simulink model "HSM_4p6U10_Motion_v01_06022022_NEW_ECC_2019a"  (R2019a)
settings: Solver=ode1  StartTime=0.0  StopTime=Inf  FixedStep=Ts  RelTol=1e-3  EnableMultiTasking=on
PostLoadFcn:
  | , if any(exist('dsrtsu_mdlpostloadfcn', 'file') == [2, 3, 6]), try dsrtsu_mdlpostloadfcn('Execute', bdroot); catch fprintf('Error in PostLoadFcn (dsrtsu_mdlpostloadfcn) for model "%s":\n %s\n', bdroot, lasterr); end, end,
values from neighbouring files (symbols this model uses):
  CDP = -1    [Parameters_4p6U10.m]
  CUP = 1    [Parameters_4p6U10.m]
  HDP = 1    [Parameters_4p6U10.m]
  HUP = -1    [Parameters_4p6U10.m]
  K1m = 1.7E-4    (= 0.00017)    [Parameters_4p6U10.m]
  K2m = 7.0E-4    (= 0.0007)    [Parameters_4p6U10.m]
  Ts = 0.0002    [Parameters_4p6U10.m]
undefined symbols (not defined in the file or in its folder): GPTRIP1SEL, GPTRIP2SEL, TZ1, TZ2
libraries: simulink_extras x25, simulink x17, c2837xDlib x11, c2802xlib x2, idelinklib_common x1
(part 1 of 3)
PreSaveFcn:
  | , if any(exist('dsmpb_private', 'file') == [2, 3, 6]), try, dsmpb_private('dsmpb_mdlclblib', 'PreSave', bdroot); catch, disp(lasterr); end, end,
CloseFcn:
  | , if any(exist('dsmpb_private', 'file') == [2, 3, 6]), try, dsmpb_private('dsmpb_mdlclblib', 'Close', bdroot); catch, disp(lasterr); end, end,
settings Model: DSRTSU_INTERNAL_RTI_VER=500  DSRTSU_INTERNAL_RTI_TYPE=rti1007  DSRTSU_INTERNAL_RTIFPGA=90  DSMPB_DATASERVER_ModelPortLibVersion1=8  DSMPB_DATASERVER_DataServerVersion1=6  DSMPB_DATASERVER_DataServerStreamVersion1=3  SimulationMode=external  ExtModeTrigDuration=8  Creator=Christos  LastModifiedBy=ThermoLift
settings DataIOCC: ReturnWorkspaceOutputs=off
settings OptimizationCC: BlockReduction=off  ConditionallyExecuteInputs=off  DefaultParameterBehavior=Inlined  DefaultUnderspecifiedDataType=single  StrengthReduction=on  PassReuseOutputArgsAs=Individual arguments  MaxStackSize=512  OptimizeBlockOrder=speed
settings DebuggingCC: AlgebraicLoopMsg=none  ArtificialAlgebraicLoopMsg=none  ParameterPrecisionLossMsg=none  ParameterTunabilityLossMsg=error  SFUnexpectedBacktrackingDiag=warning  SFNoUnconditionalDefaultTransitionDiag=warning  SFExecutionAtInitializationDiag=none  ArithmeticOperatorsInVariantConditions=warning
settings HardwareCC: ProdBitPerChar=16  ProdBitPerInt=16  ProdBitPerPointer=32  ProdBitPerSizeT=32  ProdBitPerPtrDiffT=32  ProdLargestAtomicInteger=Integer  ProdLargestAtomicFloat=None  ProdWordSize=16  ProdHWDeviceType=Texas Instruments->C2000  TargetIntDivRoundTo=Zero  TargetEndianess=BigEndian  TargetHWDeviceType=Custom Processor->Custom
settings SFSimCC: SimUseLocalCustomCode=off  MATLABDynamicMemAlloc=off
settings RTWCC: SystemTargetFile=ert.tlc  HardwareBoard=TI Delfino F28379D LaunchPad  TLCOptions=-aInlineSetEventsForThisBaseRateFcn=TLC_FALSE -aSuppressMultiTaskScheduler=TLC_FALSE -aRateBasedStepFcn=1  TemplateMakefile=ert_default_tmf  GenerateReport=on  RTWUseLocalCustomCode=off  Toolchain=Texas Instruments Code Composer Studio (C2000)  IncludeHyperlinkInReport=on  LaunchReport=on  GenerateTraceInfo=on  GenerateTraceReport=on  GenerateTraceReportSl=on  GenerateTraceReportSf=on  GenerateTraceReportEml=on
settings CodeAppCC: ForceParamTrailComments=on  IgnoreCustomStorageClasses=off  OperatorAnnotations=on  SimulinkDataObjDesc=on  SFDataObjDesc=on  InsertBlockDesc=on  StateflowObjectComments=on
settings ERTTargetCC: CodeReplacementLibrary=TI C28x  SupportContinuousTime=on
settings ConfigComp: CovMetricSettings=dw  CovHtmlReporting=on  CovSaveCumulativeToWorkspaceVar=on  CovSaveSingleToWorkspaceVar=on  CovExternalEMLEnable=off
settings SimscapeCC: SimscapeNormalizeSystem=off

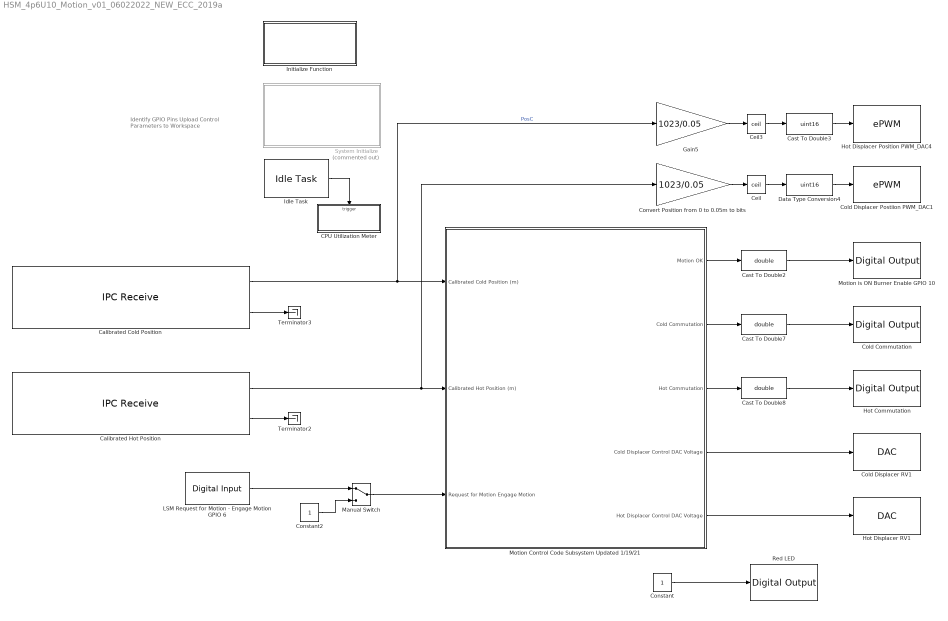
== system HSM_4p6U10_Motion_v01_06022022_NEW_ECC_2019a ==
  note: Identify GPIO Pins
      | Upload Control Parameters to Workspace
  CPU Utilization Meter : Subsystem  TreatAsAtomicUnit=on
  "Calibrated Cold Position " : c2837xDlib/IPC Receive  SelectChannel=0  DataType=single  DataLength=1  EnableBlocking=off  SampleTime=Ts
      settings: SourceProductName=Embedded Coder Support Package for Texas Instruments C2000 Processors  SourceProductBaseCode=TIC2000
  Calibrated Hot Position : c2837xDlib/IPC Receive  SelectChannel=1  DataType=single  DataLength=1  EnableBlocking=off  SampleTime=Ts
      settings: SourceProductName=Embedded Coder Support Package for Texas Instruments C2000 Processors  SourceProductBaseCode=TIC2000
  Cast To Double2 : DataTypeConversion  OutDataTypeStr=double
  Cast To Double3 : DataTypeConversion  OutDataTypeStr=uint16
  Cast To Double7 : DataTypeConversion  OutDataTypeStr=double
  Cast To Double8 : DataTypeConversion  OutDataTypeStr=double
  Ceil : Rounding  Operator=ceil
  Ceil3 : Rounding  Operator=ceil
  Cold Commutation : c2837xDlib/Digital Output  GPIO_Number=GPIO24~GPIO31  GPIO_Bit0=off  GPIO_BIT0_Toggle=off  GPIO_Bit1=off  GPIO_BIT1_Toggle=off  GPIO_Bit2=off  GPIO_BIT2_Toggle=off  GPIO_Bit3=on  GPIO_BIT3_Toggle=off  GPIO_Bit4=off  GPIO_BIT4_Toggle=off  GPIO_Bit5=off  GPIO_BIT5_Toggle=off  GPIO_Bit6=off  GPIO_BIT6_Toggle=off  GPIO_Bit7=off  GPIO_BIT7_Toggle=off
      settings: SourceProductName=Embedded Coder Support Package for Texas Instruments C2000 Processors  SourceProductBaseCode=TIC2000
  Cold Displacer Postiion PWM_DAC1 : c2802xlib/ePWM  useModule=ePWM6  ePWMxLINKTBPRD=Not Linked  periodUnits=Clock cycles  timerSource=Specify via dialog  timerPeriod_clk=1023  timerPeriod_sec=0.0001  tbshadow=Counter equals to zero  countingMode=Up  phaseActiveEnable=Disable  phaseDirection=Count down after sync  phaseActive=0  synchronizationEnable=off  dcaevt1Sync=off  dcbevt1Sync=off  synchronizationOption=Disable  clockPrescale=1  HSclockPrescale=1  enswap=off  ePWMxAStatus=off  ePWMxAactionLogic1=Do nothing  ePWMxAactionLogic2=Set  ePWMxAactionLogic3=Clear  ePWMxAactionLogic4=Set  ePWMxAactionLogic5=Do nothing  ePWMxAactionLogic6=Do nothing  ePWMxALoadMode=Load on counter equals to zero (CTR=Zero)  ePWMxACSFenable=off  ePWMxACSFvalue=Forcing disable  ePWMxASFreload=Zero  ePWMxBStatus=on  ePWMxBactionLogic1=Do nothing  ePWMxBactionLogic2=Set  ePWMxBactionLogic3=Do nothing  ePWMxBactionLogic4=Do nothing  ePWMxBactionLogic5=Clear  ePWMxBactionLogic6=Set  ePWMxBLoadMode=Load on counter equals to zero (CTR=Zero)  ePWMxBCSFenable=off  ePWMxBCSFvalue=Forcing disable  ePWMxBSFreload=Zero  ePWNxBOutWay=off  ePWMxLINKCMPA=Not Linked  CMPAUnits=Clock cycles  CMPASource=Input port  CMPAValue_per=50  CMPAValue_clk=0  enCMPAshadow=Counter equals to zero  ePWMxLINKCMPB=Not Linked  CMPBUnits=Clock cycles  CMPBSource=Specify via dialog  CMPBValue_per=50  CMPBValue_clk=0  enCMPBshadow=Counter equals to zero  ePWMxLINKCMPC=Not Linked  CMPCUnits=Clock cycles  CMPCSource=Specify via dialog  CMPCValue_per=50  CMPCValue_clk=0  enCMPCshadow=Counter equals to zero  ePWMxLINKCMPD=Not Linked  CMPDUnits=Clock cycles  CMPDSource=Specify via dialog  CMPDValue_per=50  CMPDValue_clk=0  enCMPDshadow=Counter equals to zero  enableDBePWMxA=off  enableDBePWMxB=off  enhalfcycle=off  DBpolarity=Active high (AH)  DBedgeDelay=Positive  DBSource_ePWMxA=ePWMxA  DBSource_ePWMxB=ePWMxA  DBperiodSource=Specify via dialog  REDperiod=0  FEDperiod=0  adcstartModuleA=off  adcrequestEventA=First event  adcstartEventA=Digital Compare Module A Event 1 start of conversion (DCAEVT1.soc)  adcstartEventA_type2=Digital Compare Module A Event 1 start of conversion (DCAEVT1.soc)  adcstartModuleB=off  adcrequestEventB=First event  adcstartEventB=Counter equals to zero (CTR=Zero)  adcstartEventB_type2=Counter equals to zero (CTR=Zero)  intEn=off  intPrd=First event  intSel=Counter equals to zero (CTR=Zero)  intSel_type2=Counter equals to zero (CTR=Zero)  hrpe=off  enHRPWM=off  HRPWM_LoadMode=Counter equals to period (CTR=PRD)  HRPWM_CTLMode=Duty or Period control mode  HRPWM_EDGMode=Both edge  hrpeb=off  enHRPWMB=off  HRPWM_LoadModeB=Counter equals to zero (CTR=ZERO)  HRPWM_CTLModeB=Duty or Period control mode  HRPWM_EDGModeB=Both edge  enSFO=on  enautoconv=on  chopperEnable=off  chopperFrequency=1  chopperFirstwidth=1  chopperDuty=12.5%  tripZonesource=Specify via dialog  tzselOSHT1=off  tzselOSHT2=off  tzselOSHT3=off  tzselOSHDCAEV1=off  tzselOSHDCBEV1=off  tzselCBC1=off  tzselCBC2=off  tzselCBC3=off  tzselCBCDCAEV2=off  tzselCBCDCBEV2=off  tzselOSHT4=off  tzselOSHT5=off  tzselOSHT6=off  tzselCBC4=off  tzselCBC5=off  tzselCBC6=off  enTzOstIntr=off  enTzCbcIntr=off  enTzDCAEVT1Intr=off  enTzDCAEVT2Intr=off  enTzDCBEVT1Intr=off  enTzDCBEVT2Intr=off  ePWMxAforced=No action  ePWMxBforced=No action  DCAEVT1forced=No action  DCBEVT1forced=No action  DCAEVT2forced=No action  DCBEVT2forced=No action  dcah=Trip Zone 1 input (TZ1)  dcal=Trip Zone 2 input (TZ2)  dcbh=Trip Zone 1 input (TZ1)  dcbl=Trip Zone 2 input (TZ2)  dcah_type2=GPTRIP1SEL/(TZ1)  dcal_type2=GPTRIP2SEL/(TZ2)  dcbh_type2=GPTRIP1SEL/(TZ1)  dcbl_type2=GPTRIP2SEL/(TZ2)  gendcaevt1=Event disabled  gendcaevt2=Event disabled  gendcbevt1=Event disabled  gendcbevt2=Event disabled  dcaevt1src=DCAEVT1 with sync  dcaevt2src=DCAEVT2 with sync  dcbevt1src=DCBEVT1 with sync  dcbevt2src=DCBEVT2 with sync  pulsesel=Counter equals to zero (CTR=Zero)  blankinv=off  blankoffset=0  blankwidth=0  evsrcsel=Filtered version of DCAEVT1 (DCAEVT1FILT)  encape=off  PwmType=C2000_Type4
      settings: SourceProductName=Embedded Coder Support Package for Texas Instruments C2000 Processors
  Cold Displacer RV1 : c2837xDlib/DAC  channel=B  saturate=on
      settings: SourceProductName=Embedded Coder Support Package for Texas Instruments C2000 Processors  SourceProductBaseCode=TIC2000
  Constant : Constant  OutDataTypeStr=boolean
  Constant2 : Constant  OutDataTypeStr=boolean
  Convert Position from 0 to 0.05m to bits : Gain  Gain=1023/0.05
  Data Type Conversion4 : DataTypeConversion  OutDataTypeStr=uint16
  Gain5 : Gain  Gain=1023/0.05
  Hot Commutation : c2837xDlib/Digital Output  GPIO_Number=GPIO24~GPIO31  GPIO_Bit0=off  GPIO_BIT0_Toggle=off  GPIO_Bit1=on  GPIO_BIT1_Toggle=off  GPIO_Bit2=off  GPIO_BIT2_Toggle=off  GPIO_Bit3=off  GPIO_BIT3_Toggle=off  GPIO_Bit4=off  GPIO_BIT4_Toggle=off  GPIO_Bit5=off  GPIO_BIT5_Toggle=off  GPIO_Bit6=off  GPIO_BIT6_Toggle=off  GPIO_Bit7=off  GPIO_BIT7_Toggle=off
      settings: SourceProductName=Embedded Coder Support Package for Texas Instruments C2000 Processors  SourceProductBaseCode=TIC2000
  Hot Displacer Position PWM_DAC4 : c2802xlib/ePWM  useModule=ePWM5  ePWMxLINKTBPRD=Not Linked  periodUnits=Clock cycles  timerSource=Specify via dialog  timerPeriod_clk=1023  timerPeriod_sec=0.0001  tbshadow=Counter equals to zero  countingMode=Up  phaseActiveEnable=Disable  phaseDirection=Count down after sync  phaseActive=0  synchronizationEnable=off  dcaevt1Sync=off  dcbevt1Sync=off  synchronizationOption=Disable  clockPrescale=1  HSclockPrescale=1  enswap=off  ePWMxAStatus=on  ePWMxAactionLogic1=Do nothing  ePWMxAactionLogic2=Set  ePWMxAactionLogic3=Clear  ePWMxAactionLogic4=Set  ePWMxAactionLogic5=Do nothing  ePWMxAactionLogic6=Do nothing  ePWMxALoadMode=Load on counter equals to zero (CTR=Zero)  ePWMxACSFenable=off  ePWMxACSFvalue=Forcing disable  ePWMxASFreload=Zero  ePWMxBStatus=off  ePWMxBactionLogic1=Do nothing  ePWMxBactionLogic2=Set  ePWMxBactionLogic3=Do nothing  ePWMxBactionLogic4=Do nothing  ePWMxBactionLogic5=Clear  ePWMxBactionLogic6=Set  ePWMxBLoadMode=Load on counter equals to zero (CTR=Zero)  ePWMxBCSFenable=off  ePWMxBCSFvalue=Forcing disable  ePWMxBSFreload=Zero  ePWNxBOutWay=off  ePWMxLINKCMPA=Not Linked  CMPAUnits=Clock cycles  CMPASource=Specify via dialog  CMPAValue_per=50  CMPAValue_clk=0  enCMPAshadow=Counter equals to zero  ePWMxLINKCMPB=Not Linked  CMPBUnits=Clock cycles  CMPBSource=Input port  CMPBValue_per=50  CMPBValue_clk=0  enCMPBshadow=Counter equals to zero  ePWMxLINKCMPC=Not Linked  CMPCUnits=Clock cycles  CMPCSource=Specify via dialog  CMPCValue_per=50  CMPCValue_clk=0  enCMPCshadow=Counter equals to zero  ePWMxLINKCMPD=Not Linked  CMPDUnits=Clock cycles  CMPDSource=Specify via dialog  CMPDValue_per=50  CMPDValue_clk=0  enCMPDshadow=Counter equals to zero  enableDBePWMxA=off  enableDBePWMxB=off  enhalfcycle=off  DBpolarity=Active high (AH)  DBedgeDelay=Positive  DBSource_ePWMxA=ePWMxA  DBSource_ePWMxB=ePWMxA  DBperiodSource=Specify via dialog  REDperiod=0  FEDperiod=0  adcstartModuleA=off  adcrequestEventA=First event  adcstartEventA=Digital Compare Module A Event 1 start of conversion (DCAEVT1.soc)  adcstartEventA_type2=Digital Compare Module A Event 1 start of conversion (DCAEVT1.soc)  adcstartModuleB=off  adcrequestEventB=First event  adcstartEventB=Counter equals to zero (CTR=Zero)  adcstartEventB_type2=Counter equals to zero (CTR=Zero)  intEn=off  intPrd=First event  intSel=Counter equals to zero (CTR=Zero)  intSel_type2=Counter equals to zero (CTR=Zero)  hrpe=off  enHRPWM=off  HRPWM_LoadMode=Counter equals to period (CTR=PRD)  HRPWM_CTLMode=Duty or Period control mode  HRPWM_EDGMode=Both edge  hrpeb=off  enHRPWMB=off  HRPWM_LoadModeB=Counter equals to zero (CTR=ZERO)  HRPWM_CTLModeB=Duty or Period control mode  HRPWM_EDGModeB=Both edge  enSFO=on  enautoconv=on  chopperEnable=off  chopperFrequency=1  chopperFirstwidth=1  chopperDuty=12.5%  tripZonesource=Specify via dialog  tzselOSHT1=off  tzselOSHT2=off  tzselOSHT3=off  tzselOSHDCAEV1=off  tzselOSHDCBEV1=off  tzselCBC1=off  tzselCBC2=off  tzselCBC3=off  tzselCBCDCAEV2=off  tzselCBCDCBEV2=off  tzselOSHT4=off  tzselOSHT5=off  tzselOSHT6=off  tzselCBC4=off  tzselCBC5=off  tzselCBC6=off  enTzOstIntr=off  enTzCbcIntr=off  enTzDCAEVT1Intr=off  enTzDCAEVT2Intr=off  enTzDCBEVT1Intr=off  enTzDCBEVT2Intr=off  ePWMxAforced=No action  ePWMxBforced=No action  DCAEVT1forced=No action  DCBEVT1forced=No action  DCAEVT2forced=No action  DCBEVT2forced=No action  dcah=Trip Zone 1 input (TZ1)  dcal=Trip Zone 2 input (TZ2)  dcbh=Trip Zone 1 input (TZ1)  dcbl=Trip Zone 2 input (TZ2)  dcah_type2=GPTRIP1SEL/(TZ1)  dcal_type2=GPTRIP2SEL/(TZ2)  dcbh_type2=GPTRIP1SEL/(TZ1)  dcbl_type2=GPTRIP2SEL/(TZ2)  gendcaevt1=Event disabled  gendcaevt2=Event disabled  gendcbevt1=Event disabled  gendcbevt2=Event disabled  dcaevt1src=DCAEVT1 with sync  dcaevt2src=DCAEVT2 with sync  dcbevt1src=DCBEVT1 with sync  dcbevt2src=DCBEVT2 with sync  pulsesel=Counter equals to zero (CTR=Zero)  blankinv=off  blankoffset=0  blankwidth=0  evsrcsel=Filtered version of DCAEVT1 (DCAEVT1FILT)  encape=off  PwmType=C2000_Type4
      settings: SourceProductName=Embedded Coder Support Package for Texas Instruments C2000 Processors
  Hot Displacer RV1 : c2837xDlib/DAC  channel=A  saturate=on
      settings: SourceProductName=Embedded Coder Support Package for Texas Instruments C2000 Processors  SourceProductBaseCode=TIC2000
  Idle Task : idelinklib_common/Idle Task  tasknumbers=[1]  taskpriorities=100017  taskpreempts=[1]  showinput=off  simPriority=0
      settings: SourceProductName=MATLAB Coder  SourceProductBaseCode=ME
  Initialize Function : Subsystem  TreatAsAtomicUnit=on
  LSM Request for Motion - Engage Motion GPIO 6 : c2837xDlib/Digital Input  GPIO_Number=GPIO0~GPIO7  GPIO_Bit0=off  GPIO_Bit1=off  GPIO_Bit2=off  GPIO_Bit3=off  GPIO_Bit4=off  GPIO_Bit5=off  GPIO_Bit6=on  GPIO_Bit7=off  sampleTime=Ts  dataType=boolean  GPIO_Bit0_Qualification=Sync to SYSCLKOUT  GPIO_Bit1_Qualification=Sync to SYSCLKOUT  GPIO_Bit2_Qualification=Sync to SYSCLKOUT  GPIO_Bit3_Qualification=Sync to SYSCLKOUT  GPIO_Bit4_Qualification=Sync to SYSCLKOUT  GPIO_Bit5_Qualification=Sync to SYSCLKOUT  GPIO_Bit6_Qualification=Sync to SYSCLKOUT  GPIO_Bit7_Qualification=Sync to SYSCLKOUT  Qualification_Period=-1
      settings: SourceProductName=Embedded Coder Support Package for Texas Instruments C2000 Processors  SourceProductBaseCode=TIC2000
  Manual Switch : ManualSwitch
  Motion Control Code Subsystem Updated 1/19/21 : Subsystem
  Motion is ON Burner Enable GPIO 10 : c2837xDlib/Digital Output  GPIO_Number=GPIO8~GPIO15  GPIO_Bit0=off  GPIO_BIT0_Toggle=off  GPIO_Bit1=off  GPIO_BIT1_Toggle=off  GPIO_Bit2=on  GPIO_BIT2_Toggle=off  GPIO_Bit3=off  GPIO_BIT3_Toggle=off  GPIO_Bit4=off  GPIO_BIT4_Toggle=off  GPIO_Bit5=off  GPIO_BIT5_Toggle=off  GPIO_Bit6=off  GPIO_BIT6_Toggle=off  GPIO_Bit7=off  GPIO_BIT7_Toggle=off
      settings: SourceProductName=Embedded Coder Support Package for Texas Instruments C2000 Processors  SourceProductBaseCode=TIC2000
  Red LED : c2837xDlib/Digital Output  GPIO_Number=GPIO120~GPIO127  GPIO_Bit0=off  GPIO_BIT0_Toggle=off  GPIO_Bit1=off  GPIO_BIT1_Toggle=off  GPIO_Bit2=on  GPIO_BIT2_Toggle=off  GPIO_Bit3=off  GPIO_BIT3_Toggle=off  GPIO_Bit4=off  GPIO_BIT4_Toggle=off  GPIO_Bit5=off  GPIO_BIT5_Toggle=off  GPIO_Bit6=off  GPIO_BIT6_Toggle=off  GPIO_Bit7=off  GPIO_BIT7_Toggle=off
      settings: SourceProductName=Embedded Coder Support Package for Texas Instruments C2000 Processors  SourceProductBaseCode=TIC2000
  System Initialize : Subsystem  Commented=on  mask(System Initialize){ShowInLibBrowser=0}
      mask prompts: ShowInLibBrowser "Simulink:masks:CustCodeMaskParam1_MP"
      settings: CopyFcn=cccopyfcn(gcb)  OpenFcn=ccopenfcn('System Initialize Function')
      mask Help: eval('feval(''rtwprivate'',''rtwhelpview'',''rtw_sys_initialize_block'')');
      mask Display: disp('System\nInitialize');
  Terminator2 : Terminator
  Terminator3 : Terminator
  wires:
  Idle Task/1 -> CPU Utilization Meter/Trigger
  "Calibrated Cold Position "/2 -> Terminator3/1
  Calibrated Hot Position/2 -> Terminator2/1
  "Calibrated Cold Position "/1 -> Gain5/1, Motion Control Code Subsystem Updated 1/19/21/1(Calibrated Cold Position (m))  "PosC"
  Motion Control Code Subsystem Updated 1/19/21/2(Cold Commutation) -> Cast To Double7/1
  Cast To Double3/1 -> Hot Displacer Position PWM_DAC4/1
  Convert Position from 0 to 0.05m to bits/1 -> Ceil/1
  Ceil3/1 -> Cast To Double3/1
  Ceil/1 -> Data Type Conversion4/1
  Data Type Conversion4/1 -> Cold Displacer Postiion PWM_DAC1/1
  Cast To Double7/1 -> Cold Commutation/1
  Motion Control Code Subsystem Updated 1/19/21/4(Cold Displacer Control DAC Voltage) -> Cold Displacer RV1/1
  Gain5/1 -> Ceil3/1
  Motion Control Code Subsystem Updated 1/19/21/1(Motion OK) -> Cast To Double2/1
  Cast To Double2/1 -> Motion is ON Burner Enable GPIO 10/1
  Motion Control Code Subsystem Updated 1/19/21/3(Hot Commutation) -> Cast To Double8/1
  Motion Control Code Subsystem Updated 1/19/21/5(Hot Displacer Control DAC Voltage) -> Hot Displacer RV1/1
  Cast To Double8/1 -> Hot Commutation/1
  Constant/1 -> Red LED/1
  Calibrated Hot Position/1 -> Convert Position from 0 to 0.05m to bits/1, Motion Control Code Subsystem Updated 1/19/21/2(Calibrated Hot Position (m))
  LSM Request for Motion - Engage Motion GPIO 6/1 -> Manual Switch/1
  Constant2/1 -> Manual Switch/2
  Manual Switch/1 -> Motion Control Code Subsystem Updated 1/19/21/3(Request for Motion Engage Motion)

== system HSM_4p6U10_Motion_v01_06022022_NEW_ECC_2019a/CPU Utilization Meter ==
  function : TriggerPort  TriggerType=function-call  VariantControl=Variant
  Avg. voltage toggle : c2837xDlib/Digital Output  GPIO_Number=GPIO16~GPIO23  GPIO_Bit0=off  GPIO_BIT0_Toggle=off  GPIO_Bit1=off  GPIO_BIT1_Toggle=on  GPIO_Bit2=off  GPIO_BIT2_Toggle=off  GPIO_Bit3=off  GPIO_BIT3_Toggle=off  GPIO_Bit4=off  GPIO_BIT4_Toggle=off  GPIO_Bit5=off  GPIO_BIT5_Toggle=off  GPIO_Bit6=on  GPIO_BIT6_Toggle=on  GPIO_Bit7=off  GPIO_BIT7_Toggle=off
      settings: SourceProductName=Embedded Coder Support Package for Texas Instruments C2000 Processors  SourceProductBaseCode=TIC2000
  toggle enable : Constant
  wires:
  toggle enable/1 -> Avg. voltage toggle/1

== system HSM_4p6U10_Motion_v01_06022022_NEW_ECC_2019a/Initialize Function ==
  Constant : Constant  OutDataTypeStr=boolean
  Enable Position Sensor Power : c2837xDlib/Digital Output  GPIO_Number=GPIO120~GPIO127  GPIO_Bit0=off  GPIO_BIT0_Toggle=off  GPIO_Bit1=off  GPIO_BIT1_Toggle=off  GPIO_Bit2=on  GPIO_BIT2_Toggle=off  GPIO_Bit3=off  GPIO_BIT3_Toggle=off  GPIO_Bit4=off  GPIO_BIT4_Toggle=off  GPIO_Bit5=off  GPIO_BIT5_Toggle=off  GPIO_Bit6=off  GPIO_BIT6_Toggle=off  GPIO_Bit7=off  GPIO_BIT7_Toggle=off
      settings: SourceProductName=Embedded Coder Support Package for Texas Instruments C2000 Processors  SourceProductBaseCode=TIC2000
  Event Listener : EventListener  DisableCoverage=on  EventName=reset
  wires:
  Constant/1 -> Enable Position Sensor Power/1

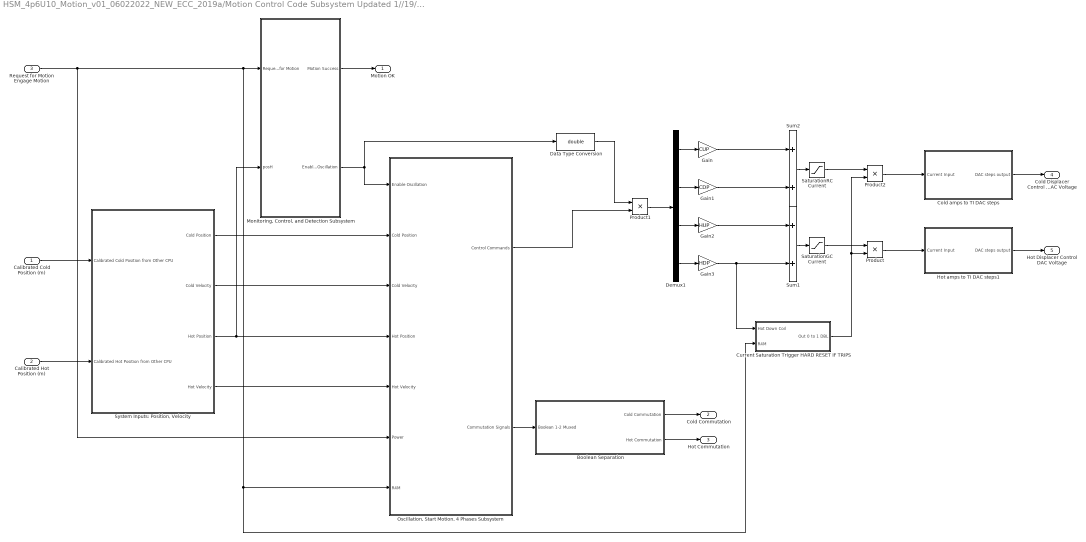
== system HSM_4p6U10_Motion_v01_06022022_NEW_ECC_2019a/Motion Control Code Subsystem Updated 1//19//21 ==
  Calibrated Cold Position (m) : Inport
  Calibrated Hot Position (m) : Inport  Port=2
  Request for Motion Engage Motion : Inport  Port=3
  Boolean Separation : Subsystem
  Cold amps to TI DAC steps : Subsystem
  Current Saturation Trigger HARD RESET IF TRIPS : Subsystem
  Data Type Conversion : DataTypeConversion  OutDataTypeStr=double
  Demux1 : Demux
  Gain : Gain  Gain=CUP
  Gain1 : Gain  Gain=CDP
  Gain2 : Gain  Gain=HUP
  Gain3 : Gain  Gain=HDP
  Hot amps to TI DAC steps1 : Subsystem
  "Monitoring, Control, and Detection Subsystem" : Subsystem
  "Oscillation, Start Motion, 4 Phases Subsystem" : Subsystem
  Product : Product
  Product1 : Product
  Product2 : Product
  SaturationGC Current : Saturate  UpperLimit=40  LowerLimit=-40
  SaturationRC Current : Saturate  UpperLimit=40  LowerLimit=-40
  Sum1 : Sum
  Sum2 : Sum
  "System Inputs: Position, Velocity" : Subsystem
  Motion OK : Outport
  Cold Commutation : Outport  Port=2
  Hot Commutation : Outport  Port=3
  Cold Displacer Control DAC Voltage : Outport  Port=4
  Hot Displacer Control DAC Voltage : Outport  Port=5
  wires:
  "Oscillation, Start Motion, 4 Phases Subsystem"/2(Commutation Signals) -> Boolean Separation/1(Boolean 1-2 Muxed)
  Calibrated Cold Position (m)/1 -> "System Inputs: Position, Velocity"/1(Calibrated Cold Position from Other CPU)
  Calibrated Hot Position (m)/1 -> "System Inputs: Position, Velocity"/2(Calibrated Hot Position from Other CPU)
  "Monitoring, Control, and Detection Subsystem"/2(Enable Oscillation) -> "Oscillation, Start Motion, 4 Phases Subsystem"/1("Enable Oscillation "), Data Type Conversion/1
  Boolean Separation/1(Cold Commutation) -> Cold Commutation/1
  Boolean Separation/2(Hot Commutation) -> Hot Commutation/1
  Hot amps to TI DAC steps1/1(DAC steps output) -> Hot Displacer Control DAC Voltage/1
  Cold amps to TI DAC steps/1("DAC steps output    ") -> Cold Displacer Control DAC Voltage/1
  "System Inputs: Position, Velocity"/1(Cold Position) -> "Oscillation, Start Motion, 4 Phases Subsystem"/2(Cold Position)
  "System Inputs: Position, Velocity"/2(Cold Velocity) -> "Oscillation, Start Motion, 4 Phases Subsystem"/3(Cold Velocity)
  "System Inputs: Position, Velocity"/3(Hot Position) -> "Oscillation, Start Motion, 4 Phases Subsystem"/4(Hot Position), "Monitoring, Control, and Detection Subsystem"/2(posH)
  "System Inputs: Position, Velocity"/4(Hot Velocity) -> "Oscillation, Start Motion, 4 Phases Subsystem"/5(Hot Velocity)
  Request for Motion Engage Motion/1 -> "Oscillation, Start Motion, 4 Phases Subsystem"/6(Power), "Oscillation, Start Motion, 4 Phases Subsystem"/7(R4M), Current Saturation Trigger HARD RESET IF TRIPS/2(R4M), "Monitoring, Control, and Detection Subsystem"/1(Request for Motion)
  "Oscillation, Start Motion, 4 Phases Subsystem"/1("Control Commands ") -> Product1/2
  Data Type Conversion/1 -> Product1/1
  "Monitoring, Control, and Detection Subsystem"/1(Motion Success) -> Motion OK/1
  Current Saturation Trigger HARD RESET IF TRIPS/1(Out 0 to 1 DBL) -> Product2/2, Product/2
  Demux1/2 -> Gain1/1
  Product1/1 -> Demux1/1
  Product/1 -> Hot amps to TI DAC steps1/1(Current Input)
  Gain/1 -> Sum2/1
  SaturationRC Current/1 -> Product2/1
  Product2/1 -> Cold amps to TI DAC steps/1(Current Input)
  Gain2/1 -> Sum1/1
  Sum1/1 -> SaturationGC Current/1
  Demux1/1 -> Gain/1
  Gain3/1 -> Sum1/2, Current Saturation Trigger HARD RESET IF TRIPS/1(Hot Down Coil)
  SaturationGC Current/1 -> Product/1
  Sum2/1 -> SaturationRC Current/1
  Gain1/1 -> Sum2/2
  Demux1/3 -> Gain2/1
  Demux1/4 -> Gain3/1

== system HSM_4p6U10_Motion_v01_06022022_NEW_ECC_2019a/System Initialize ==

== system HSM_4p6U10_Motion_v01_06022022_NEW_ECC_2019a/Motion Control Code Subsystem Updated 1//19//21/Boolean Separation ==
  Boolean 1-2 Muxed : Inport
  Data Type Conversion : DataTypeConversion  OutDataTypeStr=double
  Data Type Conversion1 : DataTypeConversion  OutDataTypeStr=double
  Demux : Demux  Outputs=2
  Gain : Gain  Gain=5
  Gain1 : Gain  Gain=5
  Cold Commutation : Outport
  Hot Commutation : Outport  Port=2
  wires:
  Demux/1 -> Data Type Conversion/1  "Q1Sep"
  Demux/2 -> Data Type Conversion1/1  "Q2Sep"
  Boolean 1-2 Muxed/1 -> Demux/1
  Data Type Conversion/1 -> Gain/1
  Data Type Conversion1/1 -> Gain1/1
  Gain/1 -> Cold Commutation/1
  Gain1/1 -> Hot Commutation/1

== system HSM_4p6U10_Motion_v01_06022022_NEW_ECC_2019a/Motion Control Code Subsystem Updated 1//19//21/Cold amps to TI DAC steps ==
  Current Input : Inport
  Add : Sum
  Amps to Voltage Servo Conversion Gain : Gain  Gain=1/6
  Shift 0 A to DAC midrange : Constant  Value=2098
  Volts to DAC steps : Gain  Gain=208.7
  "DAC steps output    " : Outport
  wires:
  Shift 0 A to DAC midrange/1 -> Add/1
  Volts to DAC steps/1 -> Add/2
  Current Input/1 -> Amps to Voltage Servo Conversion Gain/1
  Add/1 -> "DAC steps output    "/1
  Amps to Voltage Servo Conversion Gain/1 -> Volts to DAC steps/1

== system HSM_4p6U10_Motion_v01_06022022_NEW_ECC_2019a/Motion Control Code Subsystem Updated 1//19//21/Current Saturation Trigger HARD RESET IF TRIPS ==
  Hot Down Coil : Inport
  R4M : Inport  Port=2
  39p5Amps : HitCross  HitCrossingOffset=39.5  HitCrossingDirection=falling
  39p99Amps : HitCross  HitCrossingOffset=39.99  HitCrossingDirection=rising
  Abs : Abs
  Constant : Constant  OutDataTypeStr=double
  Data Type Conversion1 : DataTypeConversion  OutDataTypeStr=double
  Detect Decrease : simulink/Logic and Bit Operations/Detect Decrease  vinit=0.0  OutDataTypeStr=boolean
  Detect Increase : simulink/Logic and Bit Operations/Detect Increase  vinit=0.0  OutDataTypeStr=boolean
  Logical Operator8 : Logic  Operator=NOT  AllPortsSameDT=off  OutDataTypeStr=boolean
  Manual Switch : ManualSwitch  CurrentSetting=0
  Reset : Subsystem
  S-R Flip-Flop : simulink_extras/Flip Flops/S-R Flip-Flop  initial_condition=0
  S-R Flip-Flop1 : simulink_extras/Flip Flops/S-R Flip-Flop  initial_condition=0
  S-R Flip-Flop2 : simulink_extras/Flip Flops/S-R Flip-Flop  initial_condition=0
  Sat Limit : simulink/Logic and Bit Operations/Compare To Constant  relop=>  const=2  OutDataTypeStr=boolean
  Terminator : Terminator
  Terminator1 : Terminator
  Terminator2 : Terminator
  Timer : Subsystem
  Out 0 to 1 DBL : Outport
  wires:
  S-R Flip-Flop1/1 -> Logical Operator8/1
  S-R Flip-Flop/2 -> Terminator1/1
  Logical Operator8/1 -> Data Type Conversion1/1
  Sat Limit/1 -> S-R Flip-Flop1/1  "Coil Timing Trigger"
  39p5Amps/1 -> S-R Flip-Flop/2
  S-R Flip-Flop/1 -> Timer/Enable
  Hot Down Coil/1 -> Abs/1
  39p99Amps/1 -> S-R Flip-Flop/1
  Timer/1(CST) -> Sat Limit/1
  S-R Flip-Flop1/2 -> Terminator2/1
  Data Type Conversion1/1 -> Manual Switch/2
  Abs/1 -> 39p99Amps/1, 39p5Amps/1
  Manual Switch/1 -> Out 0 to 1 DBL/1
  Constant/1 -> Manual Switch/1
  R4M/1 -> Detect Decrease/1, Detect Increase/1
  Detect Increase/1 -> S-R Flip-Flop2/1
  Detect Decrease/1 -> S-R Flip-Flop2/2
  S-R Flip-Flop2/1 -> Reset/Enable
  S-R Flip-Flop2/2 -> Terminator/1
  Reset/1(Reset 2s) -> S-R Flip-Flop1/2

== system HSM_4p6U10_Motion_v01_06022022_NEW_ECC_2019a/Motion Control Code Subsystem Updated 1//19//21/Hot amps to TI DAC steps1 ==
  Current Input : Inport
  Add : Sum
  Amps to Volts Servo Conversion Gain : Gain  Gain=1/6
  Shift 0 A to DAC midrange : Constant  Value=2099
  Volts to DAC steps : Gain  Gain=210
  DAC steps output : Outport
  wires:
  Volts to DAC steps/1 -> Add/2
  Current Input/1 -> Amps to Volts Servo Conversion Gain/1
  Shift 0 A to DAC midrange/1 -> Add/1
  Add/1 -> DAC steps output/1
  Amps to Volts Servo Conversion Gain/1 -> Volts to DAC steps/1

== system HSM_4p6U10_Motion_v01_06022022_NEW_ECC_2019a/Motion Control Code Subsystem Updated 1//19//21/Monitoring, Control, and Detection Subsystem ==
  Request for Motion : Inport
  posH : Inport  Port=2
  Logical Operator2 : Logic  Operator=NOT  AllPortsSameDT=off  OutDataTypeStr=boolean
  Logical Operator5 : Logic  Operator=OR  AllPortsSameDT=off  OutDataTypeStr=boolean
  S-R Flip-Flop : simulink_extras/Flip Flops/S-R Flip-Flop  initial_condition=0
  S-R Flip-Flop1 : simulink_extras/Flip Flops/S-R Flip-Flop  initial_condition=0
  S-R Flip-Flop2 : simulink_extras/Flip Flops/S-R Flip-Flop  initial_condition=0
  Subsystem : Subsystem
  Terminator1 : Terminator
  Terminator3 : Terminator
  Terminator5 : Terminator
  Unit Delay : UnitDelay  SampleTime=-1  HasFrameUpgradeWarning=on
  Unit Delay1 : UnitDelay  SampleTime=-1  HasFrameUpgradeWarning=on
  Motion Success : Outport
  Enable Oscillation : Outport  Port=2
  wires:
  Unit Delay1/1 -> S-R Flip-Flop1/2
  S-R Flip-Flop2/2 -> Terminator1/1
  S-R Flip-Flop2/1 -> Logical Operator5/2
  Logical Operator2/1 -> Logical Operator5/1, S-R Flip-Flop2/2, Unit Delay/1
  Subsystem/1(Motion Failure) -> S-R Flip-Flop2/1
  posH/1 -> Subsystem/2(posH)
  S-R Flip-Flop1/1 -> Motion Success/1  "Enable Start Up Part 1"
  S-R Flip-Flop/1 -> Enable Oscillation/1  "Activate Hot Oscillation,  Attempt to move  Cold Displacer toward BDC"
  Subsystem/2(Motion Success) -> S-R Flip-Flop1/1
  Request for Motion/1 -> S-R Flip-Flop/1, Subsystem/1(Power), Subsystem/3(En Osc), Logical Operator2/1
  Logical Operator5/1 -> Unit Delay1/1
  Unit Delay/1 -> S-R Flip-Flop/2
  S-R Flip-Flop/2 -> Terminator5/1
  S-R Flip-Flop1/2 -> Terminator3/1

== system HSM_4p6U10_Motion_v01_06022022_NEW_ECC_2019a/Motion Control Code Subsystem Updated 1//19//21/Oscillation, Start Motion, 4 Phases Subsystem ==
  "Enable Oscillation " : Inport
  Cold Position : Inport  Port=2
  Cold Velocity : Inport  Port=3
  Hot Position : Inport  Port=4
  Hot Velocity : Inport  Port=5
  Power : Inport  Port=6
  R4M : Inport  Port=7
  Constant : Constant  Value=0  OutDataTypeStr=boolean
  Oscillations Subsystem Time pc No Cold Damping : Subsystem
  Unit Delay : UnitDelay  SampleTime=-1  HasFrameUpgradeWarning=on
  "Control Commands " : Outport
  Commutation Signals : Outport  Port=2
  wires:
  Cold Velocity/1 -> Oscillations Subsystem Time pc No Cold Damping/5(VelC)
  Hot Velocity/1 -> Oscillations Subsystem Time pc No Cold Damping/2(VelH)
  Power/1 -> Oscillations Subsystem Time pc No Cold Damping/3(On/Off)
  Cold Position/1 -> Oscillations Subsystem Time pc No Cold Damping/4(Posc)
  Hot Position/1 -> Oscillations Subsystem Time pc No Cold Damping/1(Hot Position)
  Constant/1 -> Unit Delay/1
  R4M/1 -> Oscillations Subsystem Time pc No Cold Damping/7(R4M)
  "Enable Oscillation "/1 -> Oscillations Subsystem Time pc No Cold Damping/Enable
  Unit Delay/1 -> Oscillations Subsystem Time pc No Cold Damping/6(Enable 4 Phases)
  Oscillations Subsystem Time pc No Cold Damping/2(Commutation Signals) -> Commutation Signals/1
  Oscillations Subsystem Time pc No Cold Damping/1(Control Commands) -> "Control Commands "/1

== system HSM_4p6U10_Motion_v01_06022022_NEW_ECC_2019a/Motion Control Code Subsystem Updated 1//19//21/System Inputs: Position, Velocity ==
  Calibrated Cold Position from Other CPU : Inport
  Calibrated Hot Position from Other CPU : Inport  Port=2
  Cast To Double3 : DataTypeConversion  OutDataTypeStr=double
  Cast To Double4 : DataTypeConversion  OutDataTypeStr=double
  Divide by Ts : Gain  Gain=1/Ts
  Divide by Ts1 : Gain  Gain=1/Ts
  Saturation Cold Velocity : Saturate  UpperLimit=2.2  LowerLimit=-2.2
  Saturation Hot Velocity : Saturate  UpperLimit=2.2  LowerLimit=-2.2
  Second Order Cold Velocity Filter : TransferFcn  Denominator=[9e-8 6e-4 1 ]
  Second Order Hot Velocity Filter : TransferFcn  Denominator=[9e-8 6e-4 1 ]
  Sum2 : Sum  Inputs=+-
  Sum3 : Sum  Inputs=+-
  Unit Delay : UnitDelay  SampleTime=-1  HasFrameUpgradeWarning=on
  Unit Delay1 : UnitDelay  SampleTime=-1  HasFrameUpgradeWarning=on
  Cold Position : Outport
  Cold Velocity : Outport  Port=2
  Hot Position : Outport  Port=3
  Hot Velocity : Outport  Port=4
  wires:
  Calibrated Cold Position from Other CPU/1 -> Cast To Double3/1  "Cold_Position"
  Calibrated Hot Position from Other CPU/1 -> Cast To Double4/1  "Hot_Position"
  Unit Delay/1 -> Sum2/2
  Sum2/1 -> Divide by Ts/1
  Sum3/1 -> Divide by Ts1/1
  Divide by Ts/1 -> Second Order Cold Velocity Filter/1  "Discrete Derivative (Xt+1-Xt)/Ts"
  Saturation Cold Velocity/1 -> Cold Velocity/1  "Cold_Vel"
  Saturation Hot Velocity/1 -> Hot Velocity/1  "Hot_Vel"
  Second Order Cold Velocity Filter/1 -> Saturation Cold Velocity/1
  Second Order Hot Velocity Filter/1 -> Saturation Hot Velocity/1
  Unit Delay1/1 -> Sum3/2
  Divide by Ts1/1 -> Second Order Hot Velocity Filter/1
  Cast To Double3/1 -> Cold Position/1, Unit Delay/1, Sum2/1
  Cast To Double4/1 -> Unit Delay1/1, Hot Position/1, Sum3/1

== system HSM_4p6U10_Motion_v01_06022022_NEW_ECC_2019a/Motion Control Code Subsystem Updated 1//19//21/Current Saturation Trigger HARD RESET IF TRIPS/Reset ==
  Enable : EnablePort  StatesWhenEnabling=reset  ShowOutputPort=on
  Compare To Constant : simulink/Logic and Bit Operations/Compare To Constant  relop=<  const=2  OutDataTypeStr=boolean
  Constant : Constant
  Integrator : Integrator  ExternalReset=rising  LimitOutput=on  UpperSaturationLimit=5
  Reset 2s : Outport
  wires:
  Enable/1 -> Integrator/2
  Integrator/1 -> Compare To Constant/1
  Constant/1 -> Integrator/1
  Compare To Constant/1 -> Reset 2s/1

== system HSM_4p6U10_Motion_v01_06022022_NEW_ECC_2019a/Motion Control Code Subsystem Updated 1//19//21/Current Saturation Trigger HARD RESET IF TRIPS/Timer ==
  Enable : EnablePort  StatesWhenEnabling=reset  ShowOutputPort=on
  Constant : Constant
  Integrator : Integrator  ExternalReset=rising  LimitOutput=on  UpperSaturationLimit=2
  CST : Outport
  wires:
  Constant/1 -> Integrator/1
  Integrator/1 -> CST/1  "Coil Sat Time"
  Enable/1 -> Integrator/2

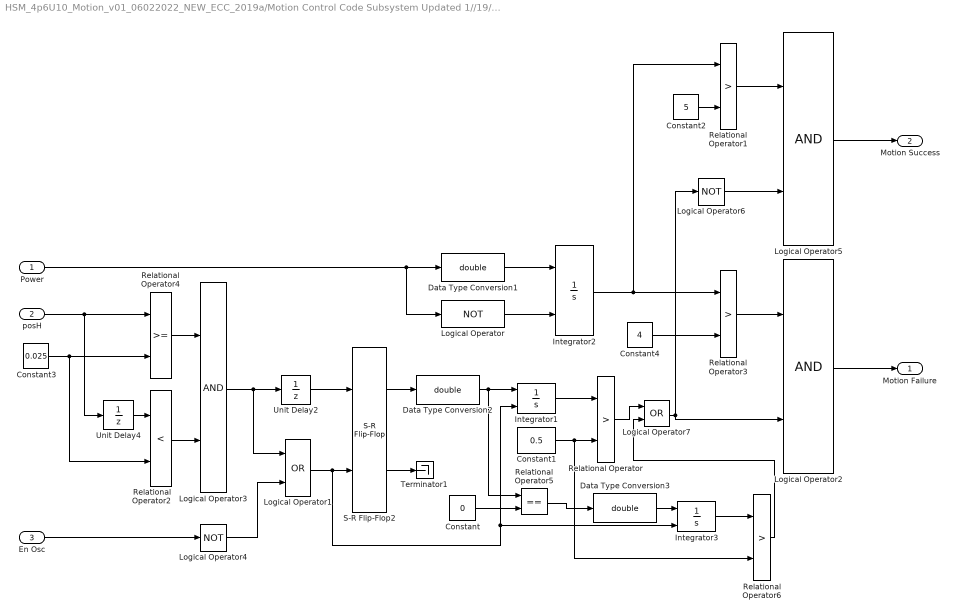
== system HSM_4p6U10_Motion_v01_06022022_NEW_ECC_2019a/Motion Control Code Subsystem Updated 1//19//21/Monitoring, Control, and Detection Subsystem/Subsystem ==
  Power : Inport
  posH : Inport  Port=2
  En Osc : Inport  Port=3
  Constant : Constant  Value=0
  Constant1 : Constant  Value=0.5
  Constant2 : Constant  Value=5
  Constant3 : Constant  Value=0.025
  Constant4 : Constant  Value=4
  Data Type Conversion1 : DataTypeConversion  OutDataTypeStr=double
  Data Type Conversion2 : DataTypeConversion  OutDataTypeStr=double
  Data Type Conversion3 : DataTypeConversion  OutDataTypeStr=double
  Integrator1 : Integrator  ExternalReset=rising  LimitOutput=on  UpperSaturationLimit=10  LowerSaturationLimit=0
  Integrator2 : Integrator  ExternalReset=level hold  LimitOutput=on  UpperSaturationLimit=20  LowerSaturationLimit=0
  Integrator3 : Integrator  ExternalReset=rising  LimitOutput=on  UpperSaturationLimit=10  LowerSaturationLimit=0
  Logical Operator : Logic  Operator=NOT  AllPortsSameDT=off  OutDataTypeStr=boolean
  Logical Operator1 : Logic  Operator=OR  AllPortsSameDT=off  OutDataTypeStr=boolean
  Logical Operator2 : Logic  AllPortsSameDT=off  OutDataTypeStr=boolean
  Logical Operator3 : Logic  AllPortsSameDT=off  OutDataTypeStr=boolean
  Logical Operator4 : Logic  Operator=NOT  AllPortsSameDT=off  OutDataTypeStr=boolean
  Logical Operator5 : Logic  AllPortsSameDT=off  OutDataTypeStr=boolean
  Logical Operator6 : Logic  Operator=NOT  AllPortsSameDT=off  OutDataTypeStr=boolean
  Logical Operator7 : Logic  Operator=OR  AllPortsSameDT=off  OutDataTypeStr=boolean
  Relational Operator{,1,3,6} (4 alike) : RelationalOperator  Operator=>  OutDataTypeStr=boolean  RndMeth=Simplest
  Relational Operator2 : RelationalOperator  Operator=<  OutDataTypeStr=boolean  RndMeth=Simplest
  Relational Operator4 : RelationalOperator  OutDataTypeStr=boolean  RndMeth=Simplest
  Relational Operator5 : RelationalOperator  Operator===  OutDataTypeStr=boolean  RndMeth=Simplest
  S-R Flip-Flop2 : simulink_extras/Flip Flops/S-R Flip-Flop  initial_condition=0
  Terminator1 : Terminator
  Unit Delay2 : UnitDelay  SampleTime=-1  HasFrameUpgradeWarning=on
  Unit Delay4 : UnitDelay  SampleTime=-1  HasFrameUpgradeWarning=on
  Motion Failure : Outport
  Motion Success : Outport  Port=2
  wires:
  S-R Flip-Flop2/1 -> Data Type Conversion2/1
  Relational Operator4/1 -> Logical Operator3/1
  posH/1 -> Relational Operator4/1, Unit Delay4/1
  Power/1 -> Logical Operator/1, Data Type Conversion1/1
  Logical Operator3/1 -> Unit Delay2/1, Logical Operator1/1
  En Osc/1 -> Logical Operator4/1
  Constant4/1 -> Relational Operator3/2
  Integrator2/1 -> Relational Operator1/1, Relational Operator3/1
  Integrator1/1 -> Relational Operator/1
  Data Type Conversion2/1 -> Relational Operator5/1, Integrator1/1
  Constant1/1 -> Relational Operator6/2, Relational Operator/2
  Unit Delay2/1 -> S-R Flip-Flop2/1
  S-R Flip-Flop2/2 -> Terminator1/1
  Logical Operator7/1 -> Logical Operator2/2, Logical Operator6/1
  Logical Operator/1 -> Integrator2/2
  Logical Operator4/1 -> Logical Operator1/2
  Logical Operator1/1 -> S-R Flip-Flop2/2, Integrator3/2, Integrator1/2
  Data Type Conversion1/1 -> Integrator2/1
  Constant3/1 -> Relational Operator4/2, Relational Operator2/2
  Relational Operator2/1 -> Logical Operator3/2
  Unit Delay4/1 -> Relational Operator2/1
  Relational Operator3/1 -> Logical Operator2/1
  Logical Operator2/1 -> Motion Failure/1
  Constant2/1 -> Relational Operator1/2
  Relational Operator1/1 -> Logical Operator5/1
  Logical Operator6/1 -> Logical Operator5/2
  Logical Operator5/1 -> Motion Success/1
  Relational Operator5/1 -> Data Type Conversion3/1
  Constant/1 -> Relational Operator5/2
  Integrator3/1 -> Relational Operator6/1
  Relational Operator/1 -> Logical Operator7/1
  Relational Operator6/1 -> Logical Operator7/2
  Data Type Conversion3/1 -> Integrator3/1

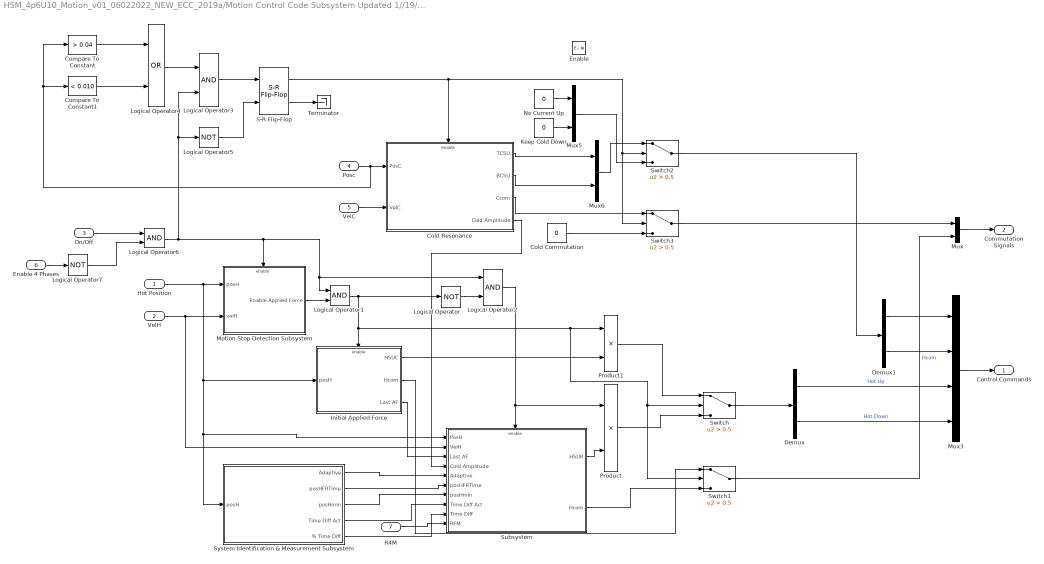
== system HSM_4p6U10_Motion_v01_06022022_NEW_ECC_2019a/Motion Control Code Subsystem Updated 1//19//21/Oscillation, Start Motion, 4 Phases Subsystem/Oscillations Subsystem Time pc No Cold Damping ==
  Hot Position : Inport
  VelH : Inport  Port=2
  On/Off : Inport  Port=3
  Posc : Inport  Port=4
  VelC : Inport  Port=5
  Enable 4 Phases : Inport  Port=6
  R4M : Inport  Port=7
  Enable : EnablePort  StatesWhenEnabling=reset
  Cold Commutation : Constant  Value=0  OutDataTypeStr=boolean
  Cold Resonance : Subsystem
  Compare To Constant : simulink/Logic and Bit Operations/Compare To Constant  relop=>  const=0.04  OutDataTypeStr=boolean
  Compare To Constant1 : simulink/Logic and Bit Operations/Compare To Constant  relop=<  const=0.010  OutDataTypeStr=boolean
  Demux : Demux  Outputs=2
  Demux1 : Demux  Outputs=2
  Initial Applied Force : Subsystem
  Keep Cold Down : Constant  Value=0
  Logical Operator : Logic  Operator=NOT  AllPortsSameDT=off  OutDataTypeStr=boolean
  Logical Operator{1..3,6} (4 alike) : Logic  AllPortsSameDT=off  OutDataTypeStr=boolean
  Logical Operator4 : Logic  Operator=OR  AllPortsSameDT=off  OutDataTypeStr=boolean
  Logical Operator5 : Logic  Operator=NOT  AllPortsSameDT=off  OutDataTypeStr=boolean
  Logical Operator7 : Logic  Operator=NOT  AllPortsSameDT=off  OutDataTypeStr=boolean
  Motion Stop Detection Subsystem : Subsystem
  Mux : Mux  Inputs=2
  Mux3 : Mux
  Mux5 : Mux  Inputs=2
  Mux6 : Mux  Inputs=2
  No Current Up : Constant  Value=0
  Product : Product
  Product1 : Product
  S-R Flip-Flop : simulink_extras/Flip Flops/S-R Flip-Flop  initial_condition=0
  Subsystem : Subsystem
  Switch{,1..3} (4 alike) : Switch  Criteria=u2 > Threshold  Threshold=0.5
  System Identification & Measurement Subsystem : Subsystem
  Terminator : Terminator
  Control Commands : Outport
  Commutation Signals : Outport  Port=2
  wires:
  Cold Resonance/4(Cold Amplitude) -> Subsystem/4(Cold Amplitude)
  Switch/1 -> Demux/1
  Enable 4 Phases/1 -> Logical Operator7/1
  Logical Operator7/1 -> Logical Operator6/2
  On/Off/1 -> Logical Operator6/1
  S-R Flip-Flop/2 -> Terminator/1
  Logical Operator5/1 -> S-R Flip-Flop/2
  Logical Operator3/1 -> S-R Flip-Flop/1
  Logical Operator4/1 -> Logical Operator3/1
  Compare To Constant1/1 -> Logical Operator4/2
  Compare To Constant/1 -> Logical Operator4/1
  Subsystem/2(Hcom) -> Switch1/3
  Product/1 -> Switch/3
  Product1/1 -> Switch/1
  Logical Operator/1 -> Logical Operator2/2
  Motion Stop Detection Subsystem/1(Enable Applied Force) -> Logical Operator1/2
  Logical Operator6/1 -> Motion Stop Detection Subsystem/Enable, Logical Operator1/1, Logical Operator2/1, Logical Operator3/2, Logical Operator5/1
  Initial Applied Force/1(HSUC) -> Product1/2
  Initial Applied Force/2(Hcom) -> Switch1/1
  Logical Operator1/1 -> Initial Applied Force/Enable, Product1/1, Switch/2, Switch1/2, Logical Operator/1
  Subsystem/1(HSUR) -> Product/2
  Hot Position/1 -> Initial Applied Force/1(posH), System Identification & Measurement Subsystem/1(posH), Subsystem/1(PosH), Motion Stop Detection Subsystem/1(posH)
  Initial Applied Force/3(Last AF) -> Subsystem/3(Last AF)
  Logical Operator2/1 -> Product/1, Subsystem/Enable
  VelH/1 -> Subsystem/2(VelH), Motion Stop Detection Subsystem/2(velH)
  VelC/1 -> Cold Resonance/2(VelC)
  Posc/1 -> Compare To Constant1/1, Compare To Constant/1, Cold Resonance/1(PosC)
  Switch2/1 -> Demux1/1
  Mux6/1 -> Switch2/1
  Cold Resonance/3(Ccom) -> Switch3/1
  Cold Resonance/2(BCSU) -> Mux6/2
  Cold Resonance/1(TCSU) -> Mux6/1
  S-R Flip-Flop/1 -> Switch3/2, Switch2/2, Cold Resonance/Enable
  Switch3/1 -> Mux/1
  Cold Commutation/1 -> Switch3/3
  Mux5/1 -> Switch2/3
  Demux1/2 -> Mux3/2
  Demux1/1 -> Mux3/1
  Switch1/1 -> Mux/2  "Hcom"
  Demux/2 -> Mux3/4  "Hot Down"
  Demux/1 -> Mux3/3  "Hot Up"
  Keep Cold Down/1 -> Mux5/2
  No Current Up/1 -> Mux5/1
  Mux/1 -> Commutation Signals/1
  Mux3/1 -> Control Commands/1
  System Identification & Measurement Subsystem/1(Adaptive) -> Subsystem/5(Adaptive)
  System Identification & Measurement Subsystem/2(posHFRTime) -> Subsystem/6(posHFRTime)
  System Identification & Measurement Subsystem/3(posHmin) -> Subsystem/7(posHmin)
  System Identification & Measurement Subsystem/4(Time Diff Act) -> Subsystem/8(Time Diff Act)
  System Identification & Measurement Subsystem/5(% Time Diff) -> Subsystem/9(Time Diff)
  R4M/1 -> Subsystem/10(RFM)

== system HSM_4p6U10_Motion_v01_06022022_NEW_ECC_2019a/Motion Control Code Subsystem Updated 1//19//21/Oscillation, Start Motion, 4 Phases Subsystem/Oscillations Subsystem Time pc No Cold Damping/Cold Resonance ==
  PosC : Inport
  VelC : Inport  Port=2
  Enable : EnablePort  ShowOutputPort=on
  Approximate Resonance Actuation : Subsystem
  Cold Down Control : Subsystem  TreatAsAtomicUnit=on
  Cold Up Control : Subsystem  TreatAsAtomicUnit=on
  Data Type Conversion : DataTypeConversion  OutDataTypeStr=double
  IBC Saturation : Saturate  UpperLimit=35  LowerLimit=0
  IRC Saturation : Saturate  UpperLimit=35  LowerLimit=0
  Product{,1..3} (4 alike) : Product
  TCSU : Outport
  BCSU : Outport  Port=2
  Ccom : Outport  Port=3
  Cold Amplitude : Outport  Port=4
  wires:
  Approximate Resonance Actuation/7(Cold Amplitude) -> Cold Amplitude/1
  Approximate Resonance Actuation/5(CDD) -> Cold Down Control/3(CDD)
  Approximate Resonance Actuation/3(CUD) -> Cold Up Control/3(CUD)
  Approximate Resonance Actuation/1(CU Activation) -> Product1/1, Cold Up Control/Enable
  Cold Up Control/1(IRC) -> IRC Saturation/1
  Data Type Conversion/1 -> Product2/1, Product3/1
  Product3/1 -> BCSU/1
  Product2/1 -> TCSU/1
  Enable/1 -> Data Type Conversion/1
  Cold Down Control/1(IBC) -> IBC Saturation/1
  Product/1 -> Product3/2
  Product1/1 -> Product2/2
  VelC/1 -> Approximate Resonance Actuation/2(VelC), Cold Up Control/1(VelC), Cold Down Control/1(VelC)
  PosC/1 -> Approximate Resonance Actuation/1(PosC), Cold Up Control/2(PosC), Cold Down Control/2(PosC)
  IBC Saturation/1 -> Product/2
  Approximate Resonance Actuation/2(CD Activation) -> Ccom/1, Product/1, Cold Down Control/Enable
  IRC Saturation/1 -> Product1/2
  Approximate Resonance Actuation/4(CUCF) -> Cold Up Control/4(CUCF)
  Approximate Resonance Actuation/6(CDCF) -> Cold Down Control/4(CDCF)

== system HSM_4p6U10_Motion_v01_06022022_NEW_ECC_2019a/Motion Control Code Subsystem Updated 1//19//21/Oscillation, Start Motion, 4 Phases Subsystem/Oscillations Subsystem Time pc No Cold Damping/Initial Applied Force ==
  posH : Inport
  Enable : EnablePort  StatesWhenEnabling=reset
  Constant : Constant  Value=0
  Constant1 : Constant  Value=0.005
  Constant2 : Constant  Value=0  OutDataTypeStr=boolean
  Constant3 : Constant  Value=0
  Constant4 : Constant
  Constant5 : Constant  OutDataTypeStr=boolean
  Grab and Hold Last Applied Force : Subsystem
  IYC Saturation : Saturate  UpperLimit=40  LowerLimit=0
  Integrator : Integrator
  Mux : Mux  Inputs=2
  N/s : Gain  Gain=-5000
  Relational Operator : RelationalOperator  Operator=<  OutDataTypeStr=boolean  RndMeth=Simplest
  Relational Operator1 : RelationalOperator  Operator=<  OutDataTypeStr=boolean  RndMeth=Simplest
  S-R Flip-Flop : simulink_extras/Flip Flops/S-R Flip-Flop  initial_condition=0
  Switch : Switch  Criteria=u2 > Threshold  Threshold=0.5
  Terminator : Terminator
  Unit Delay1 : UnitDelay  SampleTime=-1  HasFrameUpgradeWarning=on
  Unity Gain Scaling : Subsystem
  HSUC : Outport
  Hcom : Outport  Port=2
  Last AF : Outport  Port=3
  wires:
  N/s/1 -> Integrator/1
  posH/1 -> Unity Gain Scaling/2(x), Relational Operator/1
  Constant1/1 -> Relational Operator/2
  Relational Operator/1 -> S-R Flip-Flop/1
  Constant2/1 -> S-R Flip-Flop/2
  S-R Flip-Flop/2 -> Terminator/1
  Integrator/1 -> Grab and Hold Last Applied Force/1(AF), Switch/3
  Unit Delay1/1 -> Relational Operator1/1
  Relational Operator1/1 -> Grab and Hold Last Applied Force/Enable
  Grab and Hold Last Applied Force/1(Last AF) -> Last AF/1
  Constant4/1 -> N/s/1
  S-R Flip-Flop/1 -> Switch/2, Relational Operator1/2, Unit Delay1/1
  Constant3/1 -> Switch/1
  Switch/1 -> Unity Gain Scaling/1(u)  "HD Applied Force"
  Constant/1 -> Mux/1
  Constant5/1 -> Hcom/1
  Unity Gain Scaling/1(i) -> IYC Saturation/1
  Mux/1 -> HSUC/1
  IYC Saturation/1 -> Mux/2

== system HSM_4p6U10_Motion_v01_06022022_NEW_ECC_2019a/Motion Control Code Subsystem Updated 1//19//21/Oscillation, Start Motion, 4 Phases Subsystem/Oscillations Subsystem Time pc No Cold Damping/Motion Stop Detection Subsystem ==
  posH : Inport
  velH : Inport  Port=2
  Enable : EnablePort  StatesWhenEnabling=reset
  Abs : Abs
  Compare To Constant : simulink/Logic and Bit Operations/Compare To Constant  relop=>  const=0.01  OutDataTypeStr=boolean
  Constant10 : Constant  Value=0.01
  Constant2 : Constant  Value=0.015
  Constant3 : Constant  Value=0
  Data Type Conversion : DataTypeConversion  OutDataTypeStr=double
  Integrator2 : Integrator  ExternalReset=level
  Logical Operator : Logic  Operator=NOT  AllPortsSameDT=off  OutDataTypeStr=boolean
  Logical Operator1 : Logic  AllPortsSameDT=off  OutDataTypeStr=boolean
  Relational Operator1 : RelationalOperator  Operator=<  OutDataTypeStr=boolean  RndMeth=Simplest
  Relational Operator13 : RelationalOperator  Operator=<  OutDataTypeStr=boolean  RndMeth=Simplest
  Relational Operator2 : RelationalOperator  Operator=>  OutDataTypeStr=boolean  RndMeth=Simplest
  S-R Flip-Flop : simulink_extras/Flip Flops/S-R Flip-Flop  initial_condition=0
  Terminator : Terminator
  Unit Delay : UnitDelay  SampleTime=-1  HasFrameUpgradeWarning=on
  Enable Applied Force : Outport
  wires:
  Unit Delay/1 -> Enable Applied Force/1
  Logical Operator1/1 -> S-R Flip-Flop/2
  Integrator2/1 -> Compare To Constant/1
  Relational Operator13/1 -> Data Type Conversion/1, Logical Operator/1  "abs(VelH) <  0.01"
  Logical Operator/1 -> Integrator2/2
  Data Type Conversion/1 -> Integrator2/1
  Constant10/1 -> Relational Operator13/2
  Abs/1 -> Relational Operator13/1  "abs(velH)"
  Compare To Constant/1 -> S-R Flip-Flop/1  "Motion Stopped"
  Constant3/1 -> Relational Operator2/2
  Relational Operator2/1 -> Logical Operator1/2
  S-R Flip-Flop/2 -> Terminator/1
  Constant2/1 -> Relational Operator1/2
  posH/1 -> Relational Operator1/1
  Relational Operator1/1 -> Logical Operator1/1
  velH/1 -> Abs/1, Relational Operator2/1
  S-R Flip-Flop/1 -> Unit Delay/1
